simulink model "advance_compensator2_simulink"  (R2016a)
settings: Solver=VariableStepAuto  StartTime=0.0  StopTime=10.0  RelTol=1e-3
values from neighbouring files (symbols this model uses):
  Kc2 = (1)/abs(((s1+zero_cont2)/(s1+polo_cont2))*planta)    [advance_compensator.m]
  polo_cont2 = sigma + wd*tand(-deficiencia_angular - ang1)    [advance_compensator.m]
  zero_cont2 = abs(max(polos_planta))    [advance_compensator.m]
settings Model: Creator=jessa  LastModifiedBy=jessa

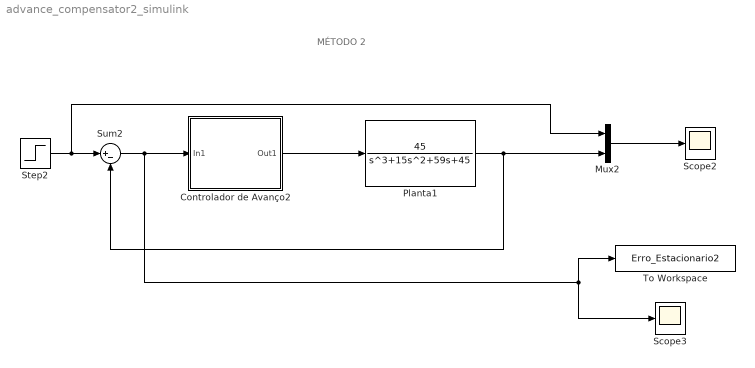
== system advance_compensator2_simulink ==
  note: MÉTODO 2
  Controlador de Avanço2 : Subsystem
  Mux2 : Mux  Inputs=2
  Planta1 : TransferFcn  Numerator=[45]  Denominator=[1 15 59 45]
  Scope2 : Scope
  Scope3 : Scope
  Step2 : Step  Time=0  SampleTime=0
  Sum2 : Sum  Inputs=|+-
  To Workspace : ToWorkspace  VariableName=Erro_Estacionario2  SampleTime=-1
  wires:
  Mux2/1 -> Scope2/1
  Planta1/1 -> Sum2/2, Mux2/2
  Step2/1 -> Sum2/1, Mux2/1
  Controlador de Avanço2/1(Out1) -> Planta1/1
  Sum2/1 -> Scope3/1, To Workspace/1, Controlador de Avanço2/1(In1)

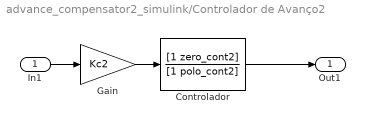
== system advance_compensator2_simulink/Controlador de Avanço2 ==
  In1 : Inport
  Controlador : TransferFcn  Numerator=[1 zero_cont2]  Denominator=[1 polo_cont2]
  Gain : Gain  Gain=Kc2
  Out1 : Outport
  wires:
  In1/1 -> Gain/1
  Gain/1 -> Controlador/1
  Controlador/1 -> Out1/1
